simulink model "SpeedControlTest_vDemo_TC"  (Simulink 6.6)
settings: Solver=ode4  SolverMode=SingleTasking  StartTime=0.0  StopTime=252  FixedStep=0.01  RelTol=1e-3
InitFcn:
  | tempomat_para
StopFcn:
  | clear;
values from neighbouring files (symbols this model uses):
  A = 1.9    [tempomat_para.m]
  a_Fzg_max = 2    [tempomat_para.m]
  a_Fzg_min = -2    [tempomat_para.m]
  cw = 0.32    [tempomat_para.m]
  gang = [1 2 3 4]    [tempomat_para.m]
  gang_vec = [1 2 3 4]    [tempomat_para.m]
  i_anteil = 5    [tempomat_para.m]
  i_d = 3.42    [tempomat_para.m]
  i_g = [3.91 2.17 1.37 1.00]    [tempomat_para.m]
  lambda_gang = [1.3 1.25  1.17  1.05]    [tempomat_para.m]
  m_Fzg = 1400    [tempomat_para.m]
  M_mot_max = [130 149 163 170 168 166 162 158 150 139 123 80]    [tempomat_para.m]
  M_mot_min = [0 -40]    [tempomat_para.m]
  n_mot0 = 1000    [tempomat_para.m]
  n_mot_max = 1000:500:6500    [tempomat_para.m]
  n_mot_min = [1000 6500]    [tempomat_para.m]
  p_anteil = 100    [tempomat_para.m]
  r_dyn = 0.28    [tempomat_para.m]
  rho = 1.202    [tempomat_para.m]
  t_sch = 0.2    [tempomat_para.m]
  TI = [block '/TI']    [PSTI_callback.m]
  v_Fzg_ms0 = 0    [tempomat_para.m]
undefined symbols (not defined in the file or in its folder): Drossel_mat, getdatatypespecs
libraries: simulink x113, fzgbib x3
(part 6 of 9)

== system SpeedControlTest_vDemo_TC/Validation Functions/R1 Speed Control step response/Complete step & CC active + no target & Speed Control active/PS/TI/Delays1 ==
  In1 : Inport
  Delay : Constant  Value=0
  Integer Delay : S-Function  FunctionName=sfix_udelay  Parameters=samptime,vinit,NumDelays,1,1,0  mask(Integer Delay){vinit=0.0, samptime=-1, NumDelays=15}
      mask prompts: vinit "Initial condition:"; samptime "Sample time:"; NumDelays "Number of delays:"
      mask help: Delay a signal N sample periods.
      mask init:
      | if isempty(NumDelays)
      |    NumDelays = 1;
      | end
      mask Display: fprintf(' %d\nZ   ',-1*(NumDelays))
  Switch : Switch  Criteria=u2 ~= 0
  Out1 : Outport
  wires:
  Integer Delay/1 -> Switch/1
  Delay/1 -> Switch/2
  In1/1 -> Integer Delay/1, Switch/3
  Switch/1 -> Out1/1

== system SpeedControlTest_vDemo_TC/Validation Functions/R1 Speed Control step response/Complete step & CC active + no target & Speed Control active/PS/TI/Delays2 ==
  In1 : Inport
  Delay : Constant  Value=0
  Integer Delay : S-Function  FunctionName=sfix_udelay  Parameters=samptime,vinit,NumDelays,1,1,0  mask(Integer Delay){vinit=0.0, samptime=-1, NumDelays=15}
      mask prompts: vinit "Initial condition:"; samptime "Sample time:"; NumDelays "Number of delays:"
      mask help: Delay a signal N sample periods.
      mask init:
      | if isempty(NumDelays)
      |    NumDelays = 1;
      | end
      mask Display: fprintf(' %d\nZ   ',-1*(NumDelays))
  Switch : Switch  Criteria=u2 ~= 0
  Out1 : Outport
  wires:
  Integer Delay/1 -> Switch/1
  Delay/1 -> Switch/2
  In1/1 -> Integer Delay/1, Switch/3
  Switch/1 -> Out1/1

== system SpeedControlTest_vDemo_TC/Validation Functions/R1 Speed Control step response/Complete step & CC active + no target & Speed Control active/PS/TID/Hold R AND1 ==
  " " : Inport
  "    " : Inport  Port=2
  Memory : Memory  Orientation=left
  Switch : Switch  Criteria=u2 ~= 0
  "  " : Outport
  wires:
  Memory/1 -> Switch/3
  Switch/1 -> Memory/1, "  "/1
  "    "/1 -> Switch/1
  " "/1 -> Switch/2

== system SpeedControlTest_vDemo_TC/Validation Functions/R1 Speed Control step response/Complete step & CC active + no target & Speed Control active/PS/TID/Hold1 ==
  " " : Inport
  "    " : Inport  Port=2
  Memory : Memory  Orientation=left
  Switch : Switch  Criteria=u2 ~= 0
  "  " : Outport
  wires:
  Memory/1 -> Switch/3
  Switch/1 -> Memory/1, "  "/1
  "    "/1 -> Switch/1
  " "/1 -> Switch/2

== system SpeedControlTest_vDemo_TC/Validation Functions/R1 Speed Control step response/Maximum overshoot < 5 &  Steady state error < 5/PAS/Delay bus signals/AD delay ==
  In1 : Inport
  Delay : Constant  Value=0
  Integer Delay : S-Function  FunctionName=sfix_udelay  Parameters=samptime,vinit,NumDelays,1,1,0  mask(Integer Delay){vinit=0.0, samptime=-1, NumDelays=15}
      mask prompts: vinit "Initial condition:"; samptime "Sample time:"; NumDelays "Number of delays:"
      mask help: Delay a signal N sample periods.
      mask init:
      | if isempty(NumDelays)
      |    NumDelays = 1;
      | end
      mask Display: fprintf(' %d\nZ   ',-1*(NumDelays))
  Switch : Switch  Criteria=u2 ~= 0
  Out1 : Outport
  wires:
  Switch/1 -> Out1/1
  In1/1 -> Switch/3, Integer Delay/1
  Delay/1 -> Switch/2
  Integer Delay/1 -> Switch/1

== system SpeedControlTest_vDemo_TC/Validation Functions/R1 Speed Control step response/Maximum overshoot < 5 &  Steady state error < 5/PAS/Delay bus signals/ELL delay ==
  In1 : Inport
  Delay : Constant  Value=0
  Integer Delay : S-Function  FunctionName=sfix_udelay  Parameters=samptime,vinit,NumDelays,1,1,0  mask(Integer Delay){vinit=0.0, samptime=-1, NumDelays=15}
      mask prompts: vinit "Initial condition:"; samptime "Sample time:"; NumDelays "Number of delays:"
      mask help: Delay a signal N sample periods.
      mask init:
      | if isempty(NumDelays)
      |    NumDelays = 1;
      | end
      mask Display: fprintf(' %d\nZ   ',-1*(NumDelays))
  Switch : Switch  Criteria=u2 ~= 0
  Out1 : Outport
  wires:
  Switch/1 -> Out1/1
  In1/1 -> Switch/3, Integer Delay/1
  Delay/1 -> Switch/2
  Integer Delay/1 -> Switch/1

== system SpeedControlTest_vDemo_TC/Validation Functions/R1 Speed Control step response/Maximum overshoot < 5 &  Steady state error < 5/PAS/Delay bus signals/EUL delay ==
  In1 : Inport
  Delay : Constant  Value=0
  Integer Delay : S-Function  FunctionName=sfix_udelay  Parameters=samptime,vinit,NumDelays,1,1,0  mask(Integer Delay){vinit=0.0, samptime=-1, NumDelays=15}
      mask prompts: vinit "Initial condition:"; samptime "Sample time:"; NumDelays "Number of delays:"
      mask help: Delay a signal N sample periods.
      mask init:
      | if isempty(NumDelays)
      |    NumDelays = 1;
      | end
      mask Display: fprintf(' %d\nZ   ',-1*(NumDelays))
  Switch : Switch  Criteria=u2 ~= 0
  Out1 : Outport
  wires:
  Integer Delay/1 -> Switch/1
  Delay/1 -> Switch/2
  In1/1 -> Integer Delay/1, Switch/3
  Switch/1 -> Out1/1

== system SpeedControlTest_vDemo_TC/Validation Functions/R1 Speed Control step response/Maximum overshoot < 5 &  Steady state error < 5/PAS/none - pass - fail/Arbitration ==
  Pass : Inport
  Fail1 : Inport  Port=2
  Fail2 : Inport  Port=3
  Fail3 : Inport  Port=4
  Fail4 : Inport  Port=5
  Delay P F1 F3 : Inport  Port=6
  Delay F2 : Inport  Port=7
  Delay F4 : Inport  Port=8
  Max delay : Inport  Port=9
  Verdict identification : Subsystem
  Verdict selection : Subsystem
  Verdict : Outport
  Delay : Outport  Port=2
  wires:
  Verdict selection/2(Delay) -> Delay/1
  Verdict selection/1(Verdict) -> Verdict/1
  Max delay/1 -> Verdict selection/6(Max delay)
  Verdict identification/2(V2) -> Verdict selection/2(V2)
  Verdict identification/1(V1) -> Verdict selection/1(V1)
  Delay F4/1 -> Verdict selection/5(Delay F4)
  Delay F2/1 -> Verdict selection/4(Delay F2)
  Delay P F1 F3/1 -> Verdict selection/3(Delay P F1 F3)
  Fail4/1 -> Verdict identification/5(Fail4)
  Fail3/1 -> Verdict identification/4(Fail3)
  Fail2/1 -> Verdict identification/3(Fail2)
  Fail1/1 -> Verdict identification/2(Fail1)
  Pass/1 -> Verdict identification/1(Pass)

== system SpeedControlTest_vDemo_TC/Validation Functions/R1 Speed Control step response/Maximum overshoot < 5 &  Steady state error < 5/PAS/none - pass - fail/Compute delay ==
  Max Delay : Inport
  R AND : Inport  Port=2
  Clock : Clock
      settings: Decimation=10
  Clock1 : Clock
      settings: Decimation=10
  Divide : Product  Inputs=/*  OutScaling=2^-10
  Hold1 : Subsystem  TreatAsAtomicUnit=on
      mask Display: patch(-0.31+[0.4 0.46 0.46 0.54 0.54 0.6 0.6 0.55 0.55 0.45 0.45 0.4],-0.19+[0.85 0.85 0.95 0.95 0.85 0.85 0.87 0.87 0.96 0.96 0.87 0.87],[0 0 0]);
  SimStepSize : Constant  Value=0.01
  Subtract : Sum  Inputs=-+  OutScaling=2^-10
  Subtract1 : Sum  Inputs=+-  OutScaling=2^-10
  Delay : Outport
  wires:
  Divide/1 -> Delay/1
  Max Delay/1 -> Subtract/1
  SimStepSize/1 -> Divide/1
  Clock/1 -> Hold1/2("    ")
  Subtract/1 -> Subtract1/2
  Subtract1/1 -> Divide/2
  Clock1/1 -> Subtract1/1
  Hold1/1("  ") -> Subtract/2
  R AND/1 -> Hold1/1(" ")

== system SpeedControlTest_vDemo_TC/Validation Functions/R1 Speed Control step response/Maximum overshoot < 5 &  Steady state error < 5/PAS/none - pass - fail/Compute delay1 ==
  Max Delay : Inport
  R AND/z : Inport  Port=2
  Add : Sum  OutScaling=2^-10
  Clock : Clock
      settings: Decimation=10
  Clock1 : Clock
      settings: Decimation=10
  Divide : Product  Inputs=/*  OutScaling=2^-10
  Hold1 : Subsystem  TreatAsAtomicUnit=on
      mask Display: patch(-0.31+[0.4 0.46 0.46 0.54 0.54 0.6 0.6 0.55 0.55 0.45 0.45 0.4],-0.19+[0.85 0.85 0.95 0.95 0.85 0.85 0.87 0.87 0.96 0.96 0.87 0.87],[0 0 0]);
  SimStepSize : Constant  Value=0.01
  Subtract : Sum  Inputs=-+  OutScaling=2^-10
  Subtract1 : Sum  Inputs=+-  OutScaling=2^-10
  Unit : Constant
  Delay : Outport
  wires:
  Divide/1 -> Add/2
  Unit/1 -> Add/1
  Max Delay/1 -> Subtract/1
  SimStepSize/1 -> Divide/1
  Clock/1 -> Hold1/2("    ")
  Subtract/1 -> Subtract1/2
  Subtract1/1 -> Divide/2
  Clock1/1 -> Subtract1/1
  Hold1/1("  ") -> Subtract/2
  R AND/z/1 -> Hold1/1(" ")
  Add/1 -> Delay/1

== system SpeedControlTest_vDemo_TC/Validation Functions/R1 Speed Control step response/Maximum overshoot < 5 &  Steady state error < 5/PAS/none - pass - fail/Compute delay2 ==
  Max Delay : Inport
  Rp & NOT(Ra) : Inport  Port=2
  Clock : Clock
      settings: Decimation=10
  Clock1 : Clock
      settings: Decimation=10
  Divide : Product  Inputs=/*  OutScaling=2^-10
  Hold1 : Subsystem  TreatAsAtomicUnit=on
      mask Display: patch(-0.31+[0.4 0.46 0.46 0.54 0.54 0.6 0.6 0.55 0.55 0.45 0.45 0.4],-0.19+[0.85 0.85 0.95 0.95 0.85 0.85 0.87 0.87 0.96 0.96 0.87 0.87],[0 0 0]);
  SimStepSize : Constant  Value=0.01
  Subtract : Sum  Inputs=-+  OutScaling=2^-10
  Subtract1 : Sum  Inputs=+-  OutScaling=2^-10
  Delay : Outport
  wires:
  Divide/1 -> Delay/1
  Rp & NOT(Ra)/1 -> Hold1/1(" ")
  Hold1/1("  ") -> Subtract/2
  Clock1/1 -> Subtract1/1
  Subtract1/1 -> Divide/2
  Subtract/1 -> Subtract1/2
  Clock/1 -> Hold1/2("    ")
  SimStepSize/1 -> Divide/1
  Max Delay/1 -> Subtract/1

== system SpeedControlTest_vDemo_TC/Validation Functions/R1 Speed Control step response/Maximum overshoot < 5 &  Steady state error < 5/PAS/none - pass - fail/Hold R AND1 ==
  " " : Inport
  "    " : Inport  Port=2
  Memory : Memory  Orientation=left
  Switch : Switch  Criteria=u2 ~= 0
  "  " : Outport
  wires:
  Memory/1 -> Switch/3
  Switch/1 -> Memory/1, "  "/1
  "    "/1 -> Switch/1
  " "/1 -> Switch/2

== system SpeedControlTest_vDemo_TC/Validation Functions/R1 Speed Control step response/Maximum overshoot < 5 &  Steady state error < 5/PAS/none - pass - fail/Hold R AND2 ==
  " " : Inport
  "    " : Inport  Port=2
  Memory : Memory  Orientation=left
  Switch : Switch  Criteria=u2 ~= 0
  "  " : Outport
  wires:
  Memory/1 -> Switch/3
  Switch/1 -> Memory/1, "  "/1
  "    "/1 -> Switch/1
  " "/1 -> Switch/2

== system SpeedControlTest_vDemo_TC/Validation Functions/R1 Speed Control step response/Maximum overshoot < 5 &  Steady state error < 5/PAS/none - pass - fail/Hold R AND3 ==
  " " : Inport
  "    " : Inport  Port=2
  Memory : Memory  Orientation=left
  Switch : Switch  Criteria=u2 ~= 0
  "  " : Outport
  wires:
  " "/1 -> Switch/2
  "    "/1 -> Switch/1
  Switch/1 -> "  "/1, Memory/1
  Memory/1 -> Switch/3

== system SpeedControlTest_vDemo_TC/Validation Functions/R1 Speed Control step response/Maximum overshoot < 5 &  Steady state error < 5/PAS/none - pass - fail/Hold1 ==
  " " : Inport
  "    " : Inport  Port=2
  Memory : Memory  Orientation=left
  Switch : Switch  Criteria=u2 ~= 0
  "  " : Outport
  wires:
  Memory/1 -> Switch/3
  Switch/1 -> Memory/1, "  "/1
  "    "/1 -> Switch/1
  " "/1 -> Switch/2

== system SpeedControlTest_vDemo_TC/Validation Functions/R1 Speed Control step response/Maximum overshoot < 5 &  Steady state error < 5/PAS/none - pass - fail/Hold2 ==
  " " : Inport
  "    " : Inport  Port=2
  Memory : Memory  Orientation=left
  Switch : Switch  Criteria=u2 ~= 0
  "  " : Outport
  wires:
  Memory/1 -> Switch/3
  Switch/1 -> Memory/1, "  "/1
  "    "/1 -> Switch/1
  " "/1 -> Switch/2

== system SpeedControlTest_vDemo_TC/Validation Functions/R1 Speed Control step response/Maximum overshoot < 5 &  Steady state error < 5/PAS/none - pass - fail/Hold3 ==
  " " : Inport
  "    " : Inport  Port=2
  Memory : Memory  Orientation=left
  Switch : Switch  Criteria=u2 ~= 0
  "  " : Outport
  wires:
  " "/1 -> Switch/2
  "    "/1 -> Switch/1
  Switch/1 -> "  "/1, Memory/1
  Memory/1 -> Switch/3

== system SpeedControlTest_vDemo_TC/Validation Functions/R1 Speed Control step response/Maximum overshoot < 5 &  Steady state error < 5/PAS/none - pass - fail/Hold4 ==
  " " : Inport
  "    " : Inport  Port=2
  Memory : Memory  Orientation=left
  Switch : Switch  Criteria=u2 ~= 0
  "  " : Outport
  wires:
  Memory/1 -> Switch/3
  Switch/1 -> Memory/1, "  "/1
  "    "/1 -> Switch/1
  " "/1 -> Switch/2

== system SpeedControlTest_vDemo_TC/Validation Functions/R1 Speed Control step response/Maximum overshoot < 5 &  Steady state error < 5/PAS/none - pass - fail/Hold5 ==
  " " : Inport
  "    " : Inport  Port=2
  Memory : Memory  Orientation=left
  Switch : Switch  Criteria=u2 ~= 0
  "  " : Outport
  wires:
  " "/1 -> Switch/2
  "    "/1 -> Switch/1
  Switch/1 -> "  "/1, Memory/1
  Memory/1 -> Switch/3

== system SpeedControlTest_vDemo_TC/Validation Functions/R1 Speed Control step response/Maximum overshoot < 5 &  Steady state error < 5/PAS1/Delay bus signals/AD delay ==
  In1 : Inport
  Delay : Constant  Value=0
  Integer Delay : S-Function  FunctionName=sfix_udelay  Parameters=samptime,vinit,NumDelays,1,1,0  mask(Integer Delay){vinit=0.0, samptime=-1, NumDelays=15}
      mask prompts: vinit "Initial condition:"; samptime "Sample time:"; NumDelays "Number of delays:"
      mask help: Delay a signal N sample periods.
      mask init:
      | if isempty(NumDelays)
      |    NumDelays = 1;
      | end
      mask Display: fprintf(' %d\nZ   ',-1*(NumDelays))
  Switch : Switch  Criteria=u2 ~= 0
  Out1 : Outport
  wires:
  Integer Delay/1 -> Switch/1
  Delay/1 -> Switch/2
  In1/1 -> Integer Delay/1, Switch/3
  Switch/1 -> Out1/1

== system SpeedControlTest_vDemo_TC/Validation Functions/R1 Speed Control step response/Maximum overshoot < 5 &  Steady state error < 5/PAS1/Delay bus signals/ELL delay ==
  In1 : Inport
  Delay : Constant  Value=0
  Integer Delay : S-Function  FunctionName=sfix_udelay  Parameters=samptime,vinit,NumDelays,1,1,0  mask(Integer Delay){vinit=0.0, samptime=-1, NumDelays=15}
      mask prompts: vinit "Initial condition:"; samptime "Sample time:"; NumDelays "Number of delays:"
      mask help: Delay a signal N sample periods.
      mask init:
      | if isempty(NumDelays)
      |    NumDelays = 1;
      | end
      mask Display: fprintf(' %d\nZ   ',-1*(NumDelays))
  Switch : Switch  Criteria=u2 ~= 0
  Out1 : Outport
  wires:
  Integer Delay/1 -> Switch/1
  Delay/1 -> Switch/2
  In1/1 -> Integer Delay/1, Switch/3
  Switch/1 -> Out1/1

== system SpeedControlTest_vDemo_TC/Validation Functions/R1 Speed Control step response/Maximum overshoot < 5 &  Steady state error < 5/PAS1/Delay bus signals/EUL delay ==
  In1 : Inport
  Delay : Constant  Value=0
  Integer Delay : S-Function  FunctionName=sfix_udelay  Parameters=samptime,vinit,NumDelays,1,1,0  mask(Integer Delay){vinit=0.0, samptime=-1, NumDelays=15}
      mask prompts: vinit "Initial condition:"; samptime "Sample time:"; NumDelays "Number of delays:"
      mask help: Delay a signal N sample periods.
      mask init:
      | if isempty(NumDelays)
      |    NumDelays = 1;
      | end
      mask Display: fprintf(' %d\nZ   ',-1*(NumDelays))
  Switch : Switch  Criteria=u2 ~= 0
  Out1 : Outport
  wires:
  Switch/1 -> Out1/1
  In1/1 -> Switch/3, Integer Delay/1
  Delay/1 -> Switch/2
  Integer Delay/1 -> Switch/1

== system SpeedControlTest_vDemo_TC/Validation Functions/R1 Speed Control step response/Maximum overshoot < 5 &  Steady state error < 5/PAS1/none - pass - fail/Arbitration ==
  Pass : Inport
  Fail1 : Inport  Port=2
  Fail2 : Inport  Port=3
  Fail3 : Inport  Port=4
  Fail4 : Inport  Port=5
  Delay P F1 F3 : Inport  Port=6
  Delay F2 : Inport  Port=7
  Delay F4 : Inport  Port=8
  Max delay : Inport  Port=9
  Verdict identification : Subsystem
  Verdict selection : Subsystem
  Verdict : Outport
  Delay : Outport  Port=2
  wires:
  Pass/1 -> Verdict identification/1(Pass)
  Fail1/1 -> Verdict identification/2(Fail1)
  Fail2/1 -> Verdict identification/3(Fail2)
  Fail3/1 -> Verdict identification/4(Fail3)
  Fail4/1 -> Verdict identification/5(Fail4)
  Delay P F1 F3/1 -> Verdict selection/3(Delay P F1 F3)
  Delay F2/1 -> Verdict selection/4(Delay F2)
  Delay F4/1 -> Verdict selection/5(Delay F4)
  Verdict identification/1(V1) -> Verdict selection/1(V1)
  Verdict identification/2(V2) -> Verdict selection/2(V2)
  Max delay/1 -> Verdict selection/6(Max delay)
  Verdict selection/1(Verdict) -> Verdict/1
  Verdict selection/2(Delay) -> Delay/1

== system SpeedControlTest_vDemo_TC/Validation Functions/R1 Speed Control step response/Maximum overshoot < 5 &  Steady state error < 5/PAS1/none - pass - fail/Compute delay ==
  Max Delay : Inport
  R AND : Inport  Port=2
  Clock : Clock
      settings: Decimation=10
  Clock1 : Clock
      settings: Decimation=10
  Divide : Product  Inputs=/*  OutScaling=2^-10
  Hold1 : Subsystem  TreatAsAtomicUnit=on
      mask Display: patch(-0.31+[0.4 0.46 0.46 0.54 0.54 0.6 0.6 0.55 0.55 0.45 0.45 0.4],-0.19+[0.85 0.85 0.95 0.95 0.85 0.85 0.87 0.87 0.96 0.96 0.87 0.87],[0 0 0]);
  SimStepSize : Constant  Value=0.01
  Subtract : Sum  Inputs=-+  OutScaling=2^-10
  Subtract1 : Sum  Inputs=+-  OutScaling=2^-10
  Delay : Outport
  wires:
  R AND/1 -> Hold1/1(" ")
  Hold1/1("  ") -> Subtract/2
  Clock1/1 -> Subtract1/1
  Subtract1/1 -> Divide/2
  Subtract/1 -> Subtract1/2
  Clock/1 -> Hold1/2("    ")
  SimStepSize/1 -> Divide/1
  Max Delay/1 -> Subtract/1
  Divide/1 -> Delay/1

== system SpeedControlTest_vDemo_TC/Validation Functions/R1 Speed Control step response/Maximum overshoot < 5 &  Steady state error < 5/PAS1/none - pass - fail/Compute delay1 ==
  Max Delay : Inport
  R AND/z : Inport  Port=2
  Add : Sum  OutScaling=2^-10
  Clock : Clock
      settings: Decimation=10
  Clock1 : Clock
      settings: Decimation=10
  Divide : Product  Inputs=/*  OutScaling=2^-10
  Hold1 : Subsystem  TreatAsAtomicUnit=on
      mask Display: patch(-0.31+[0.4 0.46 0.46 0.54 0.54 0.6 0.6 0.55 0.55 0.45 0.45 0.4],-0.19+[0.85 0.85 0.95 0.95 0.85 0.85 0.87 0.87 0.96 0.96 0.87 0.87],[0 0 0]);
  SimStepSize : Constant  Value=0.01
  Subtract : Sum  Inputs=-+  OutScaling=2^-10
  Subtract1 : Sum  Inputs=+-  OutScaling=2^-10
  Unit : Constant
  Delay : Outport
  wires:
  Add/1 -> Delay/1
  R AND/z/1 -> Hold1/1(" ")
  Hold1/1("  ") -> Subtract/2
  Clock1/1 -> Subtract1/1
  Subtract1/1 -> Divide/2
  Subtract/1 -> Subtract1/2
  Clock/1 -> Hold1/2("    ")
  SimStepSize/1 -> Divide/1
  Max Delay/1 -> Subtract/1
  Unit/1 -> Add/1
  Divide/1 -> Add/2

== system SpeedControlTest_vDemo_TC/Validation Functions/R1 Speed Control step response/Maximum overshoot < 5 &  Steady state error < 5/PAS1/none - pass - fail/Compute delay2 ==
  Max Delay : Inport
  Rp & NOT(Ra) : Inport  Port=2
  Clock : Clock
      settings: Decimation=10
  Clock1 : Clock
      settings: Decimation=10
  Divide : Product  Inputs=/*  OutScaling=2^-10
  Hold1 : Subsystem  TreatAsAtomicUnit=on
      mask Display: patch(-0.31+[0.4 0.46 0.46 0.54 0.54 0.6 0.6 0.55 0.55 0.45 0.45 0.4],-0.19+[0.85 0.85 0.95 0.95 0.85 0.85 0.87 0.87 0.96 0.96 0.87 0.87],[0 0 0]);
  SimStepSize : Constant  Value=0.01
  Subtract : Sum  Inputs=-+  OutScaling=2^-10
  Subtract1 : Sum  Inputs=+-  OutScaling=2^-10
  Delay : Outport
  wires:
  Max Delay/1 -> Subtract/1
  SimStepSize/1 -> Divide/1
  Clock/1 -> Hold1/2("    ")
  Subtract/1 -> Subtract1/2
  Subtract1/1 -> Divide/2
  Clock1/1 -> Subtract1/1
  Hold1/1("  ") -> Subtract/2
  Rp & NOT(Ra)/1 -> Hold1/1(" ")
  Divide/1 -> Delay/1

== system SpeedControlTest_vDemo_TC/Validation Functions/R1 Speed Control step response/Maximum overshoot < 5 &  Steady state error < 5/PAS1/none - pass - fail/Hold R AND1 ==
  " " : Inport
  "    " : Inport  Port=2
  Memory : Memory  Orientation=left
  Switch : Switch  Criteria=u2 ~= 0
  "  " : Outport
  wires:
  " "/1 -> Switch/2
  "    "/1 -> Switch/1
  Switch/1 -> "  "/1, Memory/1
  Memory/1 -> Switch/3

== system SpeedControlTest_vDemo_TC/Validation Functions/R1 Speed Control step response/Maximum overshoot < 5 &  Steady state error < 5/PAS1/none - pass - fail/Hold R AND2 ==
  " " : Inport
  "    " : Inport  Port=2
  Memory : Memory  Orientation=left
  Switch : Switch  Criteria=u2 ~= 0
  "  " : Outport
  wires:
  " "/1 -> Switch/2
  "    "/1 -> Switch/1
  Switch/1 -> "  "/1, Memory/1
  Memory/1 -> Switch/3

== system SpeedControlTest_vDemo_TC/Validation Functions/R1 Speed Control step response/Maximum overshoot < 5 &  Steady state error < 5/PAS1/none - pass - fail/Hold R AND3 ==
  " " : Inport
  "    " : Inport  Port=2
  Memory : Memory  Orientation=left
  Switch : Switch  Criteria=u2 ~= 0
  "  " : Outport
  wires:
  Memory/1 -> Switch/3
  Switch/1 -> Memory/1, "  "/1
  "    "/1 -> Switch/1
  " "/1 -> Switch/2

== system SpeedControlTest_vDemo_TC/Validation Functions/R1 Speed Control step response/Maximum overshoot < 5 &  Steady state error < 5/PAS1/none - pass - fail/Hold1 ==
  " " : Inport
  "    " : Inport  Port=2
  Memory : Memory  Orientation=left
  Switch : Switch  Criteria=u2 ~= 0
  "  " : Outport
  wires:
  " "/1 -> Switch/2
  "    "/1 -> Switch/1
  Switch/1 -> "  "/1, Memory/1
  Memory/1 -> Switch/3

== system SpeedControlTest_vDemo_TC/Validation Functions/R1 Speed Control step response/Maximum overshoot < 5 &  Steady state error < 5/PAS1/none - pass - fail/Hold2 ==
  " " : Inport
  "    " : Inport  Port=2
  Memory : Memory  Orientation=left
  Switch : Switch  Criteria=u2 ~= 0
  "  " : Outport
  wires:
  " "/1 -> Switch/2
  "    "/1 -> Switch/1
  Switch/1 -> "  "/1, Memory/1
  Memory/1 -> Switch/3

== system SpeedControlTest_vDemo_TC/Validation Functions/R1 Speed Control step response/Maximum overshoot < 5 &  Steady state error < 5/PAS1/none - pass - fail/Hold3 ==
  " " : Inport
  "    " : Inport  Port=2
  Memory : Memory  Orientation=left
  Switch : Switch  Criteria=u2 ~= 0
  "  " : Outport
  wires:
  Memory/1 -> Switch/3
  Switch/1 -> Memory/1, "  "/1
  "    "/1 -> Switch/1
  " "/1 -> Switch/2

== system SpeedControlTest_vDemo_TC/Validation Functions/R1 Speed Control step response/Maximum overshoot < 5 &  Steady state error < 5/PAS1/none - pass - fail/Hold4 ==
  " " : Inport
  "    " : Inport  Port=2
  Memory : Memory  Orientation=left
  Switch : Switch  Criteria=u2 ~= 0
  "  " : Outport
  wires:
  " "/1 -> Switch/2
  "    "/1 -> Switch/1
  Switch/1 -> "  "/1, Memory/1
  Memory/1 -> Switch/3

== system SpeedControlTest_vDemo_TC/Validation Functions/R1 Speed Control step response/Maximum overshoot < 5 &  Steady state error < 5/PAS1/none - pass - fail/Hold5 ==
  " " : Inport
  "    " : Inport  Port=2
  Memory : Memory  Orientation=left
  Switch : Switch  Criteria=u2 ~= 0
  "  " : Outport
  wires:
  Memory/1 -> Switch/3
  Switch/1 -> Memory/1, "  "/1
  "    "/1 -> Switch/1
  " "/1 -> Switch/2

== system SpeedControlTest_vDemo_TC/Validation Functions/R1 Speed Control step response/Maximum overshoot < 5 &  Steady state error < 5/Step response characteristics/Step response characteristics extraction/Expected set point and step parameters ==
  Step/z : Inport
  Step : Inport  Port=2
  Static Gain : Inport  Port=3
  Trigger : TriggerPort
  Compare To Zero : simulink/Logic and Bit Operations/Compare To Zero  SystemSampleTime=-1  relop=>  LogicOutDataTypeMode=uint8  ZeroCross=off
  Divide : Product  Inputs=**  OutScaling=2^-10
  Divide1 : Product  Inputs=**  OutScaling=2^-10
  Subtract : Sum  Inputs=-+  OutScaling=2^-10
  Step sign : Outport
  Set point : Outport  Port=2
  Response step size : Outport  Port=3
  wires:
  Divide/1 -> Set point/1
  Static Gain/1 -> Divide/2, Divide1/2
  Step/1 -> Divide/1, Subtract/2
  Step/z/1 -> Subtract/1
  Subtract/1 -> Compare To Zero/1, Divide1/1
  Compare To Zero/1 -> Step sign/1
  Divide1/1 -> Response step size/1

== system SpeedControlTest_vDemo_TC/Validation Functions/R1 Speed Control step response/Maximum overshoot < 5 &  Steady state error < 5/Step response characteristics/Step response characteristics extraction/Extract maximum overshoot ==
  Step response : Inport
  Reset : Inport  Port=2
  Step sign : Inport  Port=3
  Active if signals constant for some specified time : Subsystem
  Detect increase : Subsystem  TreatAsAtomicUnit=on
  Detect increase1 : Subsystem  TreatAsAtomicUnit=on
  Detect increase2 : Subsystem  TreatAsAtomicUnit=on
  Hold value with counter : Subsystem  TreatAsAtomicUnit=on
  Logical Operator : Logic  Operator=OR  Inputs=3  AllPortsSameDT=off  OutDataTypeMode=Boolean
  Step response moving average and initial conditions before step : Subsystem  TreatAsAtomicUnit=on
  Subtract : Sum  Inputs=+-  OutScaling=2^-10
  Trigger hold value : Subsystem  TreatAsAtomicUnit=on
  Maximum overshoot : Outport
  wires:
  Step response moving average and initial conditions before step/1(d(Step Response) average) -> Trigger hold value/1(d(Step Response) average)
  Step response/1 -> Active if signals constant for some specified time/2(Signal 2), Active if signals constant for some specified time/1(Signal1), Subtract/2, Hold value with counter/2(Value), Step response moving average and initial conditions before step/2(Step response)
  Step sign/1 -> Trigger hold value/2(Step sign)
  Logical Operator/1 -> Hold value with counter/Trigger
  Reset/1 -> Step response moving average and initial conditions before step/1(Reset), Hold value with counter/1(Reset counter), Detect increase2/1(Signal)
  Hold value with counter/1(Held value) -> Subtract/1
  Subtract/1 -> Maximum overshoot/1
  Trigger hold value/1(Overshoot Trigger) -> Detect increase1/1(Signal)
  Active if signals constant for some specified time/1(Constant signals) -> Detect increase/1(Signal)
  Detect increase/1(Increase) -> Logical Operator/1
  Detect increase1/1(Increase) -> Logical Operator/3
  Detect increase2/1(Increase) -> Logical Operator/2

== system SpeedControlTest_vDemo_TC/Validation Functions/R1 Speed Control step response/Maximum overshoot < 5 &  Steady state error < 5/Step response characteristics/Step response characteristics extraction/Extract rise time ==
  Step response : Inport
  Reset : Inport  Port=2
  Set point : Inport  Port=3
  Response step size : Inport  Port=4
  100 % : Constant  Value=100
  "100% " : Constant  Value=100
  Add1 : Sum  Inputs=-+  OutScaling=2^-10
  Add2 : Sum  Inputs=+-  OutScaling=2^-10
  Clock : Clock
      settings: Decimation=10
  Divide : Product  Inputs=**/  OutScaling=2^-10
  Divide1 : Product  Inputs=**/  OutScaling=2^-10
  Logical Operator : Logic  Operator=XOR  AllPortsSameDT=off  OutDataTypeMode=Boolean
  Logical Operator1 : Logic  Operator=OR  AllPortsSameDT=off  OutDataTypeMode=Boolean
  Relational Operator : RelationalOperator  LogicOutDataTypeMode=Boolean
  Relational Operator2 : RelationalOperator  Operator=<=  LogicOutDataTypeMode=Boolean
  Time difference : Subsystem  TreatAsAtomicUnit=on
  lowerLim : Constant  Value=10
  upperLim : Constant  Value=90
  Rise time : Outport
  wires:
  Clock/1 -> Time difference/2(Clock)
  Step response/1 -> Relational Operator/2, Relational Operator2/1
  Time difference/1(Time difference) -> Rise time/1
  Reset/1 -> Logical Operator1/1, Time difference/1(Reset counter)
  Logical Operator/1 -> Logical Operator1/2
  Logical Operator1/1 -> Time difference/Trigger
  lowerLim/1 -> Divide/1
  upperLim/1 -> Divide1/1
  Divide1/1 -> Add2/2
  Relational Operator2/1 -> Logical Operator/2
  Relational Operator/1 -> Logical Operator/1
  "100% "/1 -> Divide/3
  100 %/1 -> Divide1/3
  Divide/1 -> Add1/1
  Add1/1 -> Relational Operator/1
  Set point/1 -> Add1/2, Add2/1
  Response step size/1 -> Divide/2, Divide1/2
  Add2/1 -> Relational Operator2/2

== system SpeedControlTest_vDemo_TC/Validation Functions/R1 Speed Control step response/Maximum overshoot < 5 &  Steady state error < 5/Step response characteristics/Step response characteristics extraction/Extract settling time ==
  Step response : Inport
  Set point : Inport  Port=2
  Reset : Inport  Port=3
  Step time : Inport  Port=4
  " 100%" : Constant  Value=100
  Abs : Abs
  Abs1 : Abs
  Add : Sum  Inputs=+-  OutScaling=2^-10
  Add3 : Sum  Inputs=+-  OutScaling=2^-10
  Clock1 : Clock
      settings: Decimation=10
  Divide2 : Product  Inputs=**/  OutScaling=2^-10
  Logical Operator : Logic  Operator=OR  AllPortsSameDT=off  OutDataTypeMode=Boolean
  Logical Operator1 : Logic  Operator=NOT  AllPortsSameDT=off  OutDataTypeMode=Boolean
  Relational Operator3 : RelationalOperator  Operator=>  LogicOutDataTypeMode=Boolean
  Set point percent : Constant  Value=5
  Time stamp : Subsystem  TreatAsAtomicUnit=on
  Settling time : Outport
  wires:
  Logical Operator/1 -> Time stamp/Trigger
  Reset/1 -> Logical Operator/1
  Logical Operator1/1 -> Logical Operator/2
  Relational Operator3/1 -> Logical Operator1/1
  Set point/1 -> Add3/2, Divide2/1
  Step response/1 -> Add3/1
  Set point percent/1 -> Divide2/2
  Add3/1 -> Abs/1
  Abs/1 -> Relational Operator3/1
  " 100%"/1 -> Divide2/3
  Divide2/1 -> Abs1/1
  Abs1/1 -> Relational Operator3/2
  Clock1/1 -> Add/1
  Add/1 -> Time stamp/1(Clock)
  Step time/1 -> Add/2
  Time stamp/1(Time) -> Settling time/1

== system SpeedControlTest_vDemo_TC/Validation Functions/R1 Speed Control step response/Maximum overshoot < 5 &  Steady state error < 5/Step response characteristics/Step response characteristics extraction/Extract steady state error ==
  Step response : Inport
  Set point : Inport  Port=2
  Subtract : Sum  Inputs=+-  OutScaling=2^-10
  Weighted Moving Average : S-Function  FunctionName=sfix_fir  Parameters=(getdatatypespecs(OutDataType,OutScaling,DblOver,0)),[DoSatur RndMeth-1],DblOver,dolog,mgainval,(getdatatypespecs(GainDataType,GainScaling,DblOver,RadixGroup)),samptime,vinit,OutputDataTypeScalingMode,GainDataTypeScalingMode  mask(Weighted Moving Average){mgainval=0.01*ones(1,100), vinit=0.0, samptime=-1, GainDataTypeScalingMode=Inherit via internal rule, GainDataType=sfix( 16 ), MatRadixGroup=Best Precision: Matrix-wise, GainScaling=2^-10, OutputDataTypeScalingMode=Inherit via internal rule, OutDataType=sfix(16), OutScaling=2^-10, LockScale=off, RndMeth=Floor, DoSatur=off}
      mask prompts: mgainval "Weights:"; vinit "Initial condition:"; samptime "Sample time:"; GainDataTypeScalingMode "Gain data type and scaling:"; GainDataType "Parameter data type:     ex. sfix(16),  uint(8), float('single')"; MatRadixGroup "Parameter scaling mode:"; GainScaling "Parameter scaling:    Slope    ex.  2^-9"; OutputDataTypeScalingMode "Output data type and scaling:"; OutDataType "Output data type:     ex.  sfix(16),  uint(8),  float('single')"; OutScaling "Output scaling:    Slope or [Slope Bias]    ex.  2^-9"; LockScale "Lock output scaling so autoscaling tool can't change it"; RndMeth "Round toward:"; DoSatur "Saturate to max or min when overflows occur"
      mask help: Output the weighted moving average of the input.
      mask init:
      | DblOver = 0;
      | dolog = 0;
      | 
      | if MatRadixGroup == 5
      |     RadixGroup = 1; % BEST_PREC_MAT
      | elseif MatRadixGroup == 4
      |     RadixGroup = 2; % BEST_PREC_COL
      | elseif MatRadixGroup == 3
      |     RadixGroup = 3; % BEST_PREC_ROW
      | elseif MatRadixGroup == 2
      |     RadixGroup = 4; % BEST_PREC_ELE
      | else
      |     RadixGroup = 0; % BEST_PREC_OFF
      | end
      mask StyleString: edit,edit,edit,popup(Specify via dialog|Inherit via internal rule),edit,popup(Use Specified Scaling|Best Precision: Element-wise|Best Precision: Row-wise|Best Precision: Column-wise|Best Precision: Matrix-wise),edit,popup(Specify via dialog|Inherit via internal rule|Inherit via back propagation),edit,edit,checkbox,popup(Zero|Nearest|Ceiling|Floor),checkbox
      mask CallbackString: |||fixptdialog(gcbh)|fixptdialog(gcbh)|fixptdialog(gcbh)||fixptdialog(gcbh)|fixptdialog(gcbh)||||
      mask TabNameString: Main,Main,Main,Parameter data types,Parameter data types,Parameter data types,Parameter data types,Signal data types,Signal data types,Signal data types,Signal data types,Signal data types,Signal data types
      mask Display:
      | fprintf(fixpt_fir_mask_data(mgainval,'dispstr'))
      | plot(fixpt_fir_mask_data(mgainval,1),fixpt_fir_mask_data(mgainval,0))
  ss error : Outport
  wires:
  Step response/1 -> Subtract/1
  Set point/1 -> Subtract/2
  Subtract/1 -> Weighted Moving Average/1
  Weighted Moving Average/1 -> ss error/1

== system SpeedControlTest_vDemo_TC/Validation Functions/R1 Speed Control step response/Maximum overshoot < 5 &  Steady state error < 5/Step response characteristics/Step response characteristics extraction/Step time ==
  Clock : Inport
  Trigger : TriggerPort
  Time : Outport
  wires:
  Clock/1 -> Time/1

== system SpeedControlTest_vDemo_TC/Validation Functions/R1 Speed Control step response/Maximum overshoot < 5 &  Steady state error < 5/Step response characteristics/Step response reset/Active if signals constant for some specified time ==
  Signal1 : Inport
  Signal 2 : Inport  Port=2
  Logical Operator1 : Logic  AllPortsSameDT=off  OutDataTypeMode=Boolean
  Min Time : Constant  Value=10
  MinMax : MinMax  Inputs=2
  Relational Operator2 : RelationalOperator  Operator=<=  LogicOutDataTypeMode=Boolean
  Switch : Switch  Criteria=u2 ~= 0
  Time since signal constant : Subsystem  TreatAsAtomicUnit=on  mask(Feature extraction block){RT=0.0001}
      mask prompts: RT "Relative tolerance in %"
      mask help: Detect if the signal value is constant (using the last two signal values) allowing for a user-defined relative deviation
      mask CallbackString:
      | if or( (str2double(get_param(gcb,'RT')) < 0), (str2double(get_param(gcb,'RT')) > 100))
      |     error(['Relative tolerance value (' get_param(gcb,'RT') ') out of range. Please give a value between 0 and 100.']);
      | else
      |     set_param([gcb '/Detect constant/Relative tolerance/Relative Tolerance'],'Value',get_param(gcb,'RT'));
      |     set_param([gcb '/Detect constant'],'RT',get_param(gcb,'RT'));
      | end
  Time since signal constant1 : Subsystem  TreatAsAtomicUnit=on  mask(Feature extraction block){RT=0.0001}
      mask prompts: RT "Relative tolerance in %"
      mask help: Detect if the signal value is constant (using the last two signal values) allowing for a user-defined relative deviation
      mask CallbackString:
      | if or( (str2double(get_param(gcb,'RT')) < 0), (str2double(get_param(gcb,'RT')) > 100))
      |     error(['Relative tolerance value (' get_param(gcb,'RT') ') out of range. Please give a value between 0 and 100.']);
      | else
      |     set_param([gcb '/Detect constant/Relative tolerance/Relative Tolerance'],'Value',get_param(gcb,'RT'));
      |     set_param([gcb '/Detect constant'],'RT',get_param(gcb,'RT'));
      | end
  Zero : Constant  Value=0
  Constant signals : Outport
  wires:
  Signal1/1 -> Time since signal constant/1(Signal)
  Signal 2/1 -> Time since signal constant1/1(Signal)
  Relational Operator2/1 -> Constant signals/1
  Min Time/1 -> Relational Operator2/1
  Switch/1 -> Relational Operator2/2
  Time since signal constant1/2(Feature) -> MinMax/2
  Time since signal constant/2(Feature) -> MinMax/1
  Time since signal constant/1(Trigger) -> Logical Operator1/1
  Time since signal constant1/1(Trigger) -> Logical Operator1/2
  MinMax/1 -> Switch/1
  Logical Operator1/1 -> Switch/2
  Zero/1 -> Switch/3

== system SpeedControlTest_vDemo_TC/Validation Functions/R1 Speed Control step response/Maximum overshoot < 5 &  Steady state error < 5/Step response characteristics/Step response reset/Step detection ==
  Signal : Inport
  Abs : Abs
  Add : Sum  Inputs=+-  OutScaling=2^-10
  Clock : Clock
      settings: Decimation=10
  Memory : Memory
  Min step size : Constant  Value=10
  Relational Operator : RelationalOperator  LogicOutDataTypeMode=Boolean
  Switch : Switch  Criteria=u2 > Threshold
  Step : Outport
  wires:
  Add/1 -> Abs/1
  Relational Operator/1 -> Step/1
  Min step size/1 -> Relational Operator/2
  Abs/1 -> Relational Operator/1
  Signal/1 -> Memory/1, Switch/3, Add/1
  Clock/1 -> Switch/2
  Memory/1 -> Switch/1
  Switch/1 -> Add/2

== system SpeedControlTest_vDemo_TC/Validation Functions/R1 Speed Control step response/Maximum overshoot < 5 &  Steady state error < 5/Step response characteristics/Step response trigger/Active if signals constant for some specified time ==
  Signal1 : Inport
  Signal 2 : Inport  Port=2
  Logical Operator1 : Logic  AllPortsSameDT=off  OutDataTypeMode=Boolean
  Min Time : Constant  Value=10
  MinMax : MinMax  Inputs=2
  Relational Operator2 : RelationalOperator  Operator=<=  LogicOutDataTypeMode=Boolean
  Switch : Switch  Criteria=u2 ~= 0
  Time since signal constant : Subsystem  TreatAsAtomicUnit=on  mask(Feature extraction block){RT=0.001}
      mask prompts: RT "Relative tolerance in %"
      mask help: Detect if the signal value is constant (using the last two signal values) allowing for a user-defined relative deviation
      mask CallbackString:
      | if or( (str2double(get_param(gcb,'RT')) < 0), (str2double(get_param(gcb,'RT')) > 100))
      |     error(['Relative tolerance value (' get_param(gcb,'RT') ') out of range. Please give a value between 0 and 100.']);
      | else
      |     set_param([gcb '/Detect constant/Relative tolerance/Relative Tolerance'],'Value',get_param(gcb,'RT'));
      |     set_param([gcb '/Detect constant'],'RT',get_param(gcb,'RT'));
      | end
  Time since signal constant1 : Subsystem  TreatAsAtomicUnit=on  mask(Feature extraction block){RT=0.001}
      mask prompts: RT "Relative tolerance in %"
      mask help: Detect if the signal value is constant (using the last two signal values) allowing for a user-defined relative deviation
      mask CallbackString:
      | if or( (str2double(get_param(gcb,'RT')) < 0), (str2double(get_param(gcb,'RT')) > 100))
      |     error(['Relative tolerance value (' get_param(gcb,'RT') ') out of range. Please give a value between 0 and 100.']);
      | else
      |     set_param([gcb '/Detect constant/Relative tolerance/Relative Tolerance'],'Value',get_param(gcb,'RT'));
      |     set_param([gcb '/Detect constant'],'RT',get_param(gcb,'RT'));
      | end
  Zero : Constant  Value=0
  Constant signals : Outport
  wires:
  Signal1/1 -> Time since signal constant/1(Signal)
  Signal 2/1 -> Time since signal constant1/1(Signal)
  Relational Operator2/1 -> Constant signals/1
  Min Time/1 -> Relational Operator2/1
  Switch/1 -> Relational Operator2/2
  Time since signal constant1/2(Feature) -> MinMax/2
  Time since signal constant/2(Feature) -> MinMax/1
  Time since signal constant/1(Trigger) -> Logical Operator1/1
  Time since signal constant1/1(Trigger) -> Logical Operator1/2
  MinMax/1 -> Switch/1
  Logical Operator1/1 -> Switch/2
  Zero/1 -> Switch/3

== system SpeedControlTest_vDemo_TC/Validation Functions/R1 Speed Control step response/Maximum overshoot < 5 &  Steady state error < 5/Step response characteristics/Step response trigger/Compare To Constant ==
  u : Inport
  Compare : RelationalOperator  Operator=<=  LogicOutDataTypeMode=Specify via dialog  ZeroCross=off  InputSameDT=on
  Constant : Constant  Value=const  OutScaling=1
  y : Outport
  wires:
  Compare/1 -> y/1
  Constant/1 -> Compare/2
  u/1 -> Compare/1

== system SpeedControlTest_vDemo_TC/Validation Functions/R1 Speed Control step response/Maximum overshoot < 5 &  Steady state error < 5/Step response characteristics/Step response trigger/Detect increase ==
  Signal : Inport
  Clock : Clock
      settings: Decimation=10
  Memory : Memory
  Relational Operator : RelationalOperator  Operator=>  LogicOutDataTypeMode=Specify via dialog
  Switch : Switch  Criteria=u2 > Threshold
  Increase : Outport
  wires:
  Switch/1 -> Relational Operator/2
  Memory/1 -> Switch/1
  Clock/1 -> Switch/2
  Relational Operator/1 -> Increase/1
  Signal/1 -> Switch/3, Memory/1, Relational Operator/1

== system SpeedControlTest_vDemo_TC/Validation Functions/R2 Speed Control velocity restoration time after simple  acceleration or deceleration/CC active + no target & Speed Control active & step of V_Des = |1|  with time periods >= 7s/PS/TI/Delays1 ==
  In1 : Inport
  Delay : Constant  Value=0
  Integer Delay : S-Function  FunctionName=sfix_udelay  Parameters=samptime,vinit,NumDelays,1,1,0  mask(Integer Delay){vinit=0.0, samptime=-1, NumDelays=15}
      mask prompts: vinit "Initial condition:"; samptime "Sample time:"; NumDelays "Number of delays:"
      mask help: Delay a signal N sample periods.
      mask init:
      | if isempty(NumDelays)
      |    NumDelays = 1;
      | end
      mask Display: fprintf(' %d\nZ   ',-1*(NumDelays))
  Switch : Switch  Criteria=u2 ~= 0
  Out1 : Outport
  wires:
  Switch/1 -> Out1/1
  In1/1 -> Switch/3, Integer Delay/1
  Delay/1 -> Switch/2
  Integer Delay/1 -> Switch/1

== system SpeedControlTest_vDemo_TC/Validation Functions/R2 Speed Control velocity restoration time after simple  acceleration or deceleration/CC active + no target & Speed Control active & step of V_Des = |1|  with time periods >= 7s/PS/TI/Delays2 ==
  In1 : Inport
  Delay : Constant  Value=0
  Integer Delay : S-Function  FunctionName=sfix_udelay  Parameters=samptime,vinit,NumDelays,1,1,0  mask(Integer Delay){vinit=0.0, samptime=-1, NumDelays=15}
      mask prompts: vinit "Initial condition:"; samptime "Sample time:"; NumDelays "Number of delays:"
      mask help: Delay a signal N sample periods.
      mask init:
      | if isempty(NumDelays)
      |    NumDelays = 1;
      | end
      mask Display: fprintf(' %d\nZ   ',-1*(NumDelays))
  Switch : Switch  Criteria=u2 ~= 0
  Out1 : Outport
  wires:
  Switch/1 -> Out1/1
  In1/1 -> Switch/3, Integer Delay/1
  Delay/1 -> Switch/2
  Integer Delay/1 -> Switch/1

== system SpeedControlTest_vDemo_TC/Validation Functions/R2 Speed Control velocity restoration time after simple  acceleration or deceleration/CC active + no target & Speed Control active & step of V_Des = |1|  with time periods >= 7s/PS/TI/Delays3 ==
  In1 : Inport
  Delay : Constant  Value=0
  Integer Delay : S-Function  FunctionName=sfix_udelay  Parameters=samptime,vinit,NumDelays,1,1,0  mask(Integer Delay){vinit=0.0, samptime=-1, NumDelays=15}
      mask prompts: vinit "Initial condition:"; samptime "Sample time:"; NumDelays "Number of delays:"
      mask help: Delay a signal N sample periods.
      mask init:
      | if isempty(NumDelays)
      |    NumDelays = 1;
      | end
      mask Display: fprintf(' %d\nZ   ',-1*(NumDelays))
  Switch : Switch  Criteria=u2 ~= 0
  Out1 : Outport
  wires:
  Switch/1 -> Out1/1
  In1/1 -> Switch/3, Integer Delay/1
  Delay/1 -> Switch/2
  Integer Delay/1 -> Switch/1

== system SpeedControlTest_vDemo_TC/Validation Functions/R2 Speed Control velocity restoration time after simple  acceleration or deceleration/CC active + no target & Speed Control active & step of V_Des = |1|  with time periods >= 7s/PS/TID/Hold ==
  " " : Inport
  "    " : Inport  Port=2
  Memory : Memory  Orientation=left
  Switch : Switch  Criteria=u2 ~= 0
  "  " : Outport
  wires:
  Memory/1 -> Switch/3
  Switch/1 -> Memory/1, "  "/1
  "    "/1 -> Switch/1
  " "/1 -> Switch/2

== system SpeedControlTest_vDemo_TC/Validation Functions/R2 Speed Control velocity restoration time after simple  acceleration or deceleration/CC active + no target & Speed Control active & step of V_Des = |1|  with time periods >= 7s/Step with step size=|1|  and time periods >= 6s detection/Step detection/Active if signals constant for some specified time ==
  Signal 2 : Inport
  Min Time : Constant  Value=6
  Relational Operator2 : RelationalOperator  Operator=<=  LogicOutDataTypeMode=Boolean
  Switch : Switch  Criteria=u2 ~= 0
  Time since signal constant1 : Subsystem  TreatAsAtomicUnit=on  mask(Feature extraction block){RT=0.0001}
      mask prompts: RT "Relative tolerance in %"
      mask help: Detect if the signal value is constant (using the last two signal values) allowing for a user-defined relative deviation
      mask CallbackString:
      | if or( (str2double(get_param(gcb,'RT')) < 0), (str2double(get_param(gcb,'RT')) > 100))
      |     error(['Relative tolerance value (' get_param(gcb,'RT') ') out of range. Please give a value between 0 and 100.']);
      | else
      |     set_param([gcb '/Detect constant/Relative tolerance/Relative Tolerance'],'Value',get_param(gcb,'RT'));
      |     set_param([gcb '/Detect constant'],'RT',get_param(gcb,'RT'));
      | end
  Zero : Constant  Value=0
  Constant signals : Outport
  wires:
  Signal 2/1 -> Time since signal constant1/1(Signal)
  Relational Operator2/1 -> Constant signals/1
  Min Time/1 -> Relational Operator2/1
  Switch/1 -> Relational Operator2/2
  Time since signal constant1/2(Feature) -> Switch/1
  Time since signal constant1/1(Trigger) -> Switch/2
  Zero/1 -> Switch/3

== system SpeedControlTest_vDemo_TC/Validation Functions/R2 Speed Control velocity restoration time after simple  acceleration or deceleration/CC active + no target & Speed Control active & step of V_Des = |1|  with time periods >= 7s/Step with step size=|1|  and time periods >= 6s detection/Step detection/Step detection ==
  Signal : Inport
  Abs : Abs
  Add : Sum  Inputs=+-  OutScaling=2^-10
  Clock : Clock
      settings: Decimation=10
  Memory : Memory
  Relational Operator : RelationalOperator  Operator===  LogicOutDataTypeMode=Boolean
  Step size : Constant
  Switch : Switch  Criteria=u2 > Threshold
  Step : Outport
  wires:
  Add/1 -> Abs/1
  Step size/1 -> Relational Operator/2
  Abs/1 -> Relational Operator/1
  Signal/1 -> Memory/1, Switch/3, Add/1
  Clock/1 -> Switch/2
  Memory/1 -> Switch/1
  Switch/1 -> Add/2
  Relational Operator/1 -> Step/1

== system SpeedControlTest_vDemo_TC/Validation Functions/R2 Speed Control velocity restoration time after simple  acceleration or deceleration/after (6 seconds)  |V_Des-V_Vhcl <= 1.4|/PAS1/Delay bus signals/AD delay ==
  In1 : Inport
  Delay : Constant  Value=0
  Integer Delay : S-Function  FunctionName=sfix_udelay  Parameters=samptime,vinit,NumDelays,1,1,0  mask(Integer Delay){vinit=0.0, samptime=-1, NumDelays=15}
      mask prompts: vinit "Initial condition:"; samptime "Sample time:"; NumDelays "Number of delays:"
      mask help: Delay a signal N sample periods.
      mask init:
      | if isempty(NumDelays)
      |    NumDelays = 1;
      | end
      mask Display: fprintf(' %d\nZ   ',-1*(NumDelays))
  Switch : Switch  Criteria=u2 ~= 0
  Out1 : Outport
  wires:
  Switch/1 -> Out1/1
  In1/1 -> Switch/3, Integer Delay/1
  Delay/1 -> Switch/2
  Integer Delay/1 -> Switch/1

== system SpeedControlTest_vDemo_TC/Validation Functions/R2 Speed Control velocity restoration time after simple  acceleration or deceleration/after (6 seconds)  |V_Des-V_Vhcl <= 1.4|/PAS1/Delay bus signals/ELL delay ==
  In1 : Inport
  Delay : Constant  Value=0
  Integer Delay : S-Function  FunctionName=sfix_udelay  Parameters=samptime,vinit,NumDelays,1,1,0  mask(Integer Delay){vinit=0.0, samptime=-1, NumDelays=15}
      mask prompts: vinit "Initial condition:"; samptime "Sample time:"; NumDelays "Number of delays:"
      mask help: Delay a signal N sample periods.
      mask init:
      | if isempty(NumDelays)
      |    NumDelays = 1;
      | end
      mask Display: fprintf(' %d\nZ   ',-1*(NumDelays))
  Switch : Switch  Criteria=u2 ~= 0
  Out1 : Outport
  wires:
  Switch/1 -> Out1/1
  In1/1 -> Switch/3, Integer Delay/1
  Delay/1 -> Switch/2
  Integer Delay/1 -> Switch/1

== system SpeedControlTest_vDemo_TC/Validation Functions/R2 Speed Control velocity restoration time after simple  acceleration or deceleration/after (6 seconds)  |V_Des-V_Vhcl <= 1.4|/PAS1/Delay bus signals/EUL delay ==
  In1 : Inport
  Delay : Constant  Value=0
  Integer Delay : S-Function  FunctionName=sfix_udelay  Parameters=samptime,vinit,NumDelays,1,1,0  mask(Integer Delay){vinit=0.0, samptime=-1, NumDelays=15}
      mask prompts: vinit "Initial condition:"; samptime "Sample time:"; NumDelays "Number of delays:"
      mask help: Delay a signal N sample periods.
      mask init:
      | if isempty(NumDelays)
      |    NumDelays = 1;
      | end
      mask Display: fprintf(' %d\nZ   ',-1*(NumDelays))
  Switch : Switch  Criteria=u2 ~= 0
  Out1 : Outport
  wires:
  Integer Delay/1 -> Switch/1
  Delay/1 -> Switch/2
  In1/1 -> Integer Delay/1, Switch/3
  Switch/1 -> Out1/1
